simulink model "sl_RobotModelo_RRR"  (R2016b)
settings: Solver=ode45  StartTime=0.0  StopTime=5  RelTol=1e-8  EnableMultiTasking=on
values from neighbouring files (symbols this model uses):
  Aa_1 = 10    [DatosSimExp_Ideal.m]    (also in DatosSimExp_RealSR.m = 0.2; desesperacion.m = 4)
  Aa_2 = 20    [DatosSimExp_Ideal.m]    (also in DatosSimExp_RealSR.m = 0.5; desesperacion.m = 1)
  Aa_3 = 5    [DatosSimExp_Ideal.m]    (also in DatosSimExp_RealSR.m = 15; desesperacion.m = 0.5)
  Ab_1 = 20    [DatosSimExp_Ideal.m]    (also in DatosSimExp_RealSR.m = 0.003; desesperacion.m = 2)
  Ab_3 = 1    [DatosSimExp_Ideal.m]    (also in DatosSimExp_RealSR.m = 20; desesperacion.m = 0.1)
  Im_cc1 = 0    [DatosSimExp_Ideal.m]    (also in DatosSimExp_RealSR.m; desesperacion.m)
  Im_cc2 = 10    [DatosSimExp_Ideal.m]    (also in DatosSimExp_RealSR.m = 500; desesperacion.m = 2)
  Im_cc3 = 8    [DatosSimExp_Ideal.m]    (also in DatosSimExp_RealSR.m = 40; desesperacion.m = 1)
  R1 = 1    [ComparativaModelo.m]    (also in desesperacion.m = 50; pruebas.m; pruebasESTIMACION.m)
  R2 = 1    [ComparativaModelo.m]    (also in desesperacion.m = 30; pruebas.m; pruebasESTIMACION.m)
  R3 = 1    [ComparativaModelo.m]    (also in desesperacion.m = 15; pruebas.m; pruebasESTIMACION.m)
  tau1 = 5    [DatosSimExp_Ideal.m]    (also in DatosSimExp_RealSR.m = 1; desesperacion.m)
  tau2 = 5    [DatosSimExp_Ideal.m]    (also in DatosSimExp_RealSR.m = 100; desesperacion.m)
  tau3 = 5    [DatosSimExp_Ideal.m]    (also in DatosSimExp_RealSR.m = 200; desesperacion.m)
  Tm = 0.001    [ComparativaModelo.m]    (also in desesperacion.m; pruebas.m; pruebasESTIMACION.m)
  wa_1 = 50    [DatosSimExp_Ideal.m]    (also in DatosSimExp_RealSR.m = 10; desesperacion.m)
  wa_2 = 5    [DatosSimExp_Ideal.m]    (also in DatosSimExp_RealSR.m = 1; desesperacion.m)
  wa_3 = 10    [DatosSimExp_Ideal.m]    (also in DatosSimExp_RealSR.m = 0.1; desesperacion.m = 3)
  wb_1 = 1    [DatosSimExp_Ideal.m]    (also in DatosSimExp_RealSR.m = 3; desesperacion.m)
  wb_3 = 3    [DatosSimExp_Ideal.m]    (also in DatosSimExp_RealSR.m = 0.5; desesperacion.m = 10)
settings Model: ExtModeTrigMode=oneshot  ExtModeArmWhenConnect=off  Creator=Manuel G. Ortega  LastModifiedBy=marrcogrova
settings DataIOCC: SaveFormat=Array  SignalLoggingSaveFormat=ModelDataLogs
settings OptimizationCC: BooleanDataType=off  ExpressionDepthLimit=2147483647  InitFltsAndDblsToZero=on  LifeSpan=inf
settings DebuggingCC: SaveWithParameterizedLinksMsg=none  UnderspecifiedInitializationDetection=Classic  MergeDetectMultiDrivingBlocksExec=none  SignalResolutionControl=TryResolveAllWithWarning  MultiTaskDSMMsg=warning  MultiTaskCondExecSysMsg=none  FcnCallInpInsideContextMsg=warning  StateNameClashWarn=warning  SFUnexpectedBacktrackingDiag=warning  SFNoUnconditionalDefaultTransitionDiag=warning  SFExecutionAtInitializationDiag=none
settings HardwareCC: ProdBitPerPointer=32  ProdBitPerSizeT=32  ProdBitPerPtrDiffT=32  ProdLargestAtomicFloat=None  ProdIntDivRoundTo=Undefined  ProdEndianess=Unspecified  ProdWordSize=32  ProdHWDeviceType=32-bit Generic  TargetUnknown=on
settings ModelReferenceCC: PropagateSignalLabelsOutOfModel=off
settings GRTTargetCC: TargetFcnLib=ansi_tfl_tmw.mat  TargetLangStandard=C89/C90 (ANSI)  GeneratePreprocessorConditionals=Disable all  CombineOutputUpdateFcns=off  GRTInterface=on
settings ConfigComp: CovMetricSettings=dw  CovHtmlReporting=on  CovSaveCumulativeToWorkspaceVar=on  CovSaveSingleToWorkspaceVar=on  CovExternalEMLEnable=off  CovSFcnEnable=off

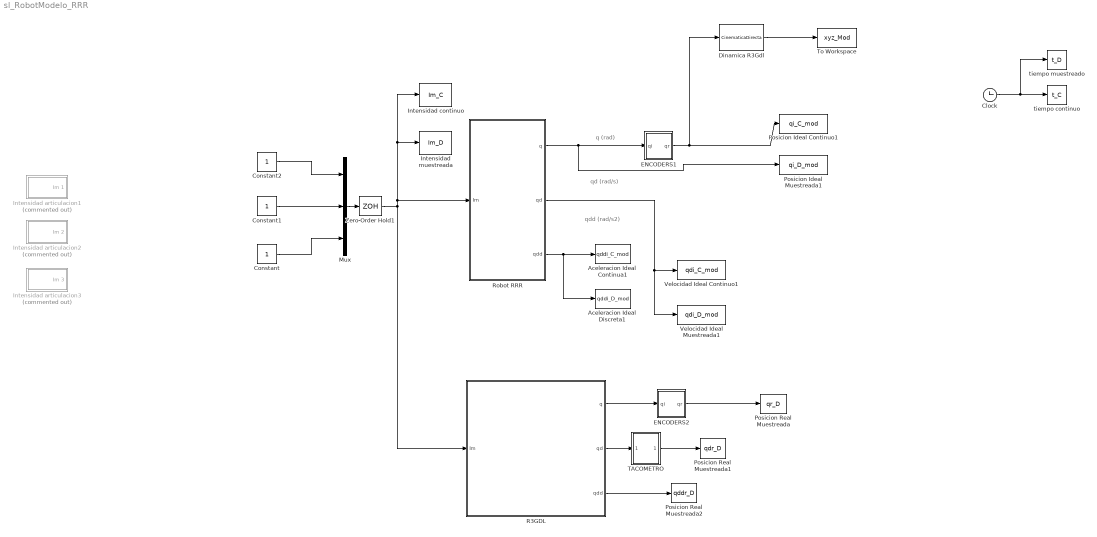
== system sl_RobotModelo_RRR ==
  note: q (rad)
  note: qd (rad/s)
  note: qdd (rad/s2)
  Aceleracion Ideal Continua1 : ToWorkspace  VariableName=qddi_C_mod  SampleTime=-1
  Aceleracion Ideal Discreta1 : ToWorkspace  VariableName=qddi_D_mod  SampleTime=Tm
  Clock : Clock
  Constant : Constant
  Constant1 : Constant
  Constant2 : Constant
  Dinamica R3Gdl : MATLABFcn  MATLABFcn=CinematicaDirecta  OutputDimensions=3
  ENCODERS1 : Subsystem
  ENCODERS2 : Subsystem
  Intensidad continuo : ToWorkspace  VariableName=Im_C  SampleTime=-1
  Intensidad articulacion1 : Subsystem  Commented=on
  Intensidad articulacion2 : Subsystem  Commented=on
  Intensidad articulacion3 : Subsystem  Commented=on
  "Intensidad muestreada " : ToWorkspace  VariableName=Im_D  SampleTime=Tm
  Mux : Mux  Inputs=3
  Posicion Ideal Continuo1 : ToWorkspace  VariableName=qi_C_mod  SampleTime=-1
  Posicion Ideal Muestreada1 : ToWorkspace  VariableName=qi_D_mod  SampleTime=Tm
  Posicion Real Muestreada : ToWorkspace  VariableName=qr_D  SampleTime=Tm
  Posicion Real Muestreada1 : ToWorkspace  VariableName=qdr_D  SampleTime=Tm
  Posicion Real Muestreada2 : ToWorkspace  VariableName=qddr_D  SampleTime=Tm
  R3GDL : Subsystem  mask(Control y Programación de Robots (4 GIERM)){NGrupo=11, q1_ini=0, q2_ini=0, q3_ini=0, Bl_q1=off, Bl_q2=off, Bl_q3=off, AccionamientoDirecto=off}
      mask prompts: NGrupo "Nº de GRUPO"; q1_ini "q1 inicial  (rad)"; q2_ini "q2 inicial (rad)"; q3_ini "q3_inicial (rad)"; Bl_q1 "Bloqueo q1"; Bl_q2 "Bloqueo q2"; Bl_q3 "Bloqueo q3"; AccionamientoDirecto "Accionamiento directo"
      mask help: Robot de 3 grados de libertad RRR
      mask Display:
      | image(imread('R3GDL_RRR.JPG'));
      | port_label('output', 1, 'q');
      | port_label('output', 2, 'qd');
      | port_label('output', 3, 'qdd');
      | port_label('input', 1, 'Im')
  Robot RRR : Subsystem
  TACOMETRO : Subsystem
  To Workspace : ToWorkspace  VariableName=xyz_Mod  SampleTime=Tm
  Velocidad Ideal Continuo1 : ToWorkspace  VariableName=qdi_C_mod  SampleTime=-1
  Velocidad Ideal Muestreada1 : ToWorkspace  VariableName=qdi_D_mod  SampleTime=Tm
  Zero-Order Hold1 : ZeroOrderHold  SampleTime=Tm
  tiempo muestreado : ToWorkspace  VariableName=t_D  SampleTime=Tm
  tiempo continuo : ToWorkspace  VariableName=t_C  SampleTime=-1
  wires:
  Clock/1 -> tiempo muestreado/1, tiempo continuo/1
  Robot RRR/3(qdd) -> Aceleracion Ideal Discreta1/1, Aceleracion Ideal Continua1/1
  Robot RRR/1(q) -> Posicion Ideal Muestreada1/1, ENCODERS1/1(qi)
  Robot RRR/2(qd) -> Velocidad Ideal Muestreada1/1, Velocidad Ideal Continuo1/1
  Dinamica R3Gdl/1 -> To Workspace/1
  Constant/1 -> Mux/3
  Constant2/1 -> Mux/1
  Constant1/1 -> Mux/2
  R3GDL/2(qd) -> TACOMETRO/1(qdi)
  R3GDL/3(qdd) -> Posicion Real Muestreada2/1
  R3GDL/1(q) -> ENCODERS2/1(qi)
  ENCODERS1/1(qr) -> Posicion Ideal Continuo1/1, Dinamica R3Gdl/1
  Mux/1 -> Zero-Order Hold1/1
  Zero-Order Hold1/1 -> Robot RRR/1(Im), "Intensidad muestreada "/1, Intensidad continuo/1, R3GDL/1(Im)
  ENCODERS2/1(qr) -> Posicion Real Muestreada/1
  TACOMETRO/1(qdr) -> Posicion Real Muestreada1/1

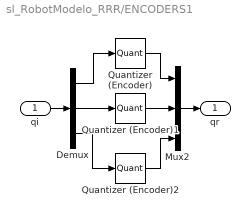
== system sl_RobotModelo_RRR/ENCODERS1 ==
  qi : Inport
  Demux : Demux  Outputs=3
  Mux2 : Mux  Inputs=3
  Quantizer (Encoder) : Quantizer  QuantizationInterval=2*pi/512/R1
  Quantizer (Encoder)1 : Quantizer  QuantizationInterval=2*pi/512/R2
  Quantizer (Encoder)2 : Quantizer  QuantizationInterval=2*pi/512/R3
  qr : Outport
  wires:
  Demux/2 -> Quantizer (Encoder)1/1
  Demux/1 -> Quantizer (Encoder)/1
  Quantizer (Encoder)1/1 -> Mux2/2
  Mux2/1 -> qr/1
  Quantizer (Encoder)2/1 -> Mux2/3
  Demux/3 -> Quantizer (Encoder)2/1
  qi/1 -> Demux/1
  Quantizer (Encoder)/1 -> Mux2/1

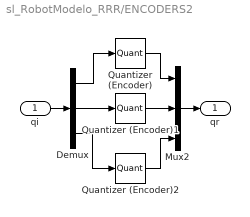
== system sl_RobotModelo_RRR/ENCODERS2 ==
  qi : Inport
  Demux : Demux  Outputs=3
  Mux2 : Mux  Inputs=3
  Quantizer (Encoder) : Quantizer  QuantizationInterval=2*pi/512/R1
  Quantizer (Encoder)1 : Quantizer  QuantizationInterval=2*pi/512/R2
  Quantizer (Encoder)2 : Quantizer  QuantizationInterval=2*pi/512/R3
  qr : Outport
  wires:
  Demux/2 -> Quantizer (Encoder)1/1
  Demux/1 -> Quantizer (Encoder)/1
  Quantizer (Encoder)1/1 -> Mux2/2
  Mux2/1 -> qr/1
  Quantizer (Encoder)2/1 -> Mux2/3
  Demux/3 -> Quantizer (Encoder)2/1
  qi/1 -> Demux/1
  Quantizer (Encoder)/1 -> Mux2/1

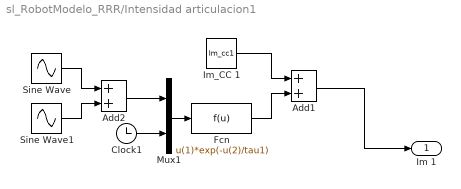
== system sl_RobotModelo_RRR/Intensidad articulacion1 ==
  Add1 : Sum
  Add2 : Sum
  Clock1 : Clock
  Fcn : Fcn  Expr=u(1)*exp(-u(2)/tau1)
  "Im_CC 1 " : Constant  Value=Im_cc1
  Mux1 : Mux  Inputs=2
  Sine Wave : Sin  Amplitude=Aa_1  Frequency=wa_1  SampleTime=0
  Sine Wave1 : Sin  Amplitude=Ab_1  Frequency=wb_1  SampleTime=0
  Im 1 : Outport
  wires:
  Add2/1 -> Mux1/1
  "Im_CC 1 "/1 -> Add1/1
  Fcn/1 -> Add1/2
  Clock1/1 -> Mux1/2
  Add1/1 -> Im 1/1
  Mux1/1 -> Fcn/1
  Sine Wave1/1 -> Add2/2
  Sine Wave/1 -> Add2/1

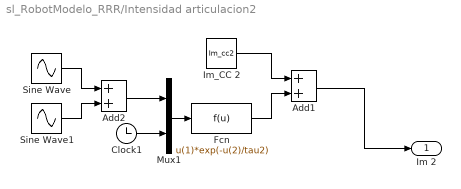
== system sl_RobotModelo_RRR/Intensidad articulacion2 ==
  Add1 : Sum
  Add2 : Sum
  Clock1 : Clock
  Fcn : Fcn  Expr=u(1)*exp(-u(2)/tau2)
  "Im_CC 2 " : Constant  Value=Im_cc2
  Mux1 : Mux  Inputs=2
  Sine Wave : Sin  Amplitude=Aa_2  Frequency=wa_2  SampleTime=0
  Sine Wave1 : Sin  Amplitude=Ab_1  Frequency=wb_1  SampleTime=0
  Im 2 : Outport
  wires:
  Add2/1 -> Mux1/1
  "Im_CC 2 "/1 -> Add1/1
  Fcn/1 -> Add1/2
  Clock1/1 -> Mux1/2
  Add1/1 -> Im 2/1
  Mux1/1 -> Fcn/1
  Sine Wave1/1 -> Add2/2
  Sine Wave/1 -> Add2/1

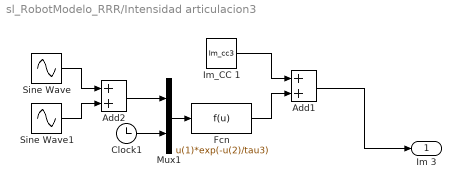
== system sl_RobotModelo_RRR/Intensidad articulacion3 ==
  Add1 : Sum
  Add2 : Sum
  Clock1 : Clock
  Fcn : Fcn  Expr=u(1)*exp(-u(2)/tau3)
  "Im_CC 1 " : Constant  Value=Im_cc3
  Mux1 : Mux  Inputs=2
  Sine Wave : Sin  Amplitude=Aa_3  Frequency=wa_3  SampleTime=0
  Sine Wave1 : Sin  Amplitude=Ab_3  Frequency=wb_3  SampleTime=0
  Im 3 : Outport
  wires:
  Add2/1 -> Mux1/1
  "Im_CC 1 "/1 -> Add1/1
  Fcn/1 -> Add1/2
  Clock1/1 -> Mux1/2
  Add1/1 -> Im 3/1
  Mux1/1 -> Fcn/1
  Sine Wave1/1 -> Add2/2
  Sine Wave/1 -> Add2/1

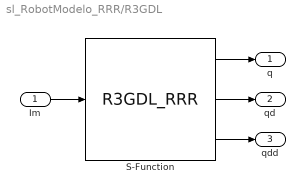
== system sl_RobotModelo_RRR/R3GDL ==
  Im : Inport
  S-Function : S-Function  FunctionName=R3GDL_RRR  Parameters=[q1_ini; q2_ini; q3_ini]; [Bl_q1; Bl_q2; Bl_q3]; AccionamientoDirecto; NGrupo  SFunctionDeploymentMode=off  EnableBusSupport=off
  q : Outport
  qd : Outport  Port=2
  qdd : Outport  Port=3
  wires:
  Im/1 -> S-Function/1
  S-Function/1 -> q/1
  S-Function/2 -> qd/1
  S-Function/3 -> qdd/1

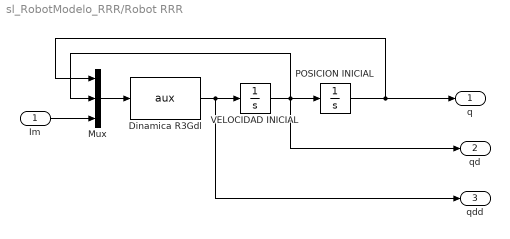
== system sl_RobotModelo_RRR/Robot RRR ==
  Im : Inport
  Dinamica R3Gdl : MATLABFcn  MATLABFcn=aux  OutputDimensions=3
  Mux : Mux  Inputs=3
  POSICION INICIAL : Integrator  InitialCondition=[0;0;0]
  VELOCIDAD INICIAL : Integrator  InitialCondition=[0;0;0];
  q : Outport
  qd : Outport  Port=2
  qdd : Outport  Port=3
  wires:
  Mux/1 -> Dinamica R3Gdl/1
  Dinamica R3Gdl/1 -> VELOCIDAD INICIAL/1, qdd/1
  VELOCIDAD INICIAL/1 -> POSICION INICIAL/1, qd/1, Mux/2
  POSICION INICIAL/1 -> q/1, Mux/1
  Im/1 -> Mux/3

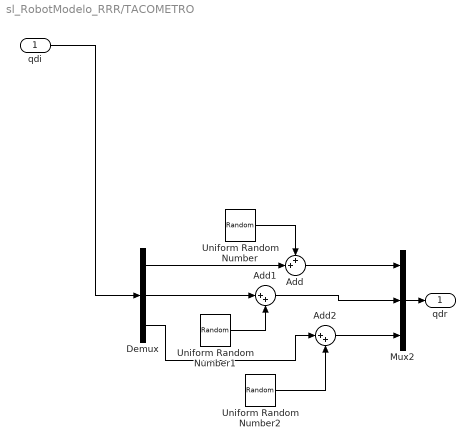
== system sl_RobotModelo_RRR/TACOMETRO ==
  qdi : Inport
  Add : Sum  Inputs=++|
  Add1 : Sum  Inputs=|++
  Add2 : Sum  Inputs=|++
  Demux : Demux  Outputs=3
  Mux2 : Mux  Inputs=3
  Uniform Random Number : UniformRandomNumber  Minimum=-(157/R1)*0.02  Maximum=(157/R1)*0.02  SampleTime=Tm
  Uniform Random Number1 : UniformRandomNumber  Minimum=-(157/R2)*0.02  Maximum=(157/R2)*0.02  SampleTime=Tm
  Uniform Random Number2 : UniformRandomNumber  Minimum=-(157/R3)*0.02  Maximum=(157/R3)*0.02  SampleTime=Tm
  qdr : Outport
  wires:
  Demux/2 -> Add1/1
  Add1/1 -> Mux2/2
  Add/1 -> Mux2/1
  Demux/1 -> Add/2
  Uniform Random Number1/1 -> Add1/2
  Add2/1 -> Mux2/3
  Uniform Random Number2/1 -> Add2/2
  Uniform Random Number/1 -> Add/1
  Demux/3 -> Add2/1
  Mux2/1 -> qdr/1
  qdi/1 -> Demux/1
